simulink model "URController"  (R2023a)
settings: Solver=ode4  StartTime=0.0  StopTime=3  FixedStep=0.001  RelTol=1e-3  EnableMultiTasking=on
values from neighbouring files (symbols this model uses):
  CYCLE_FREQ = 0.001    [init.m]
  MAX_ACC = 100    [init.m]
  MAX_VEL = 180    [init.m]
libraries: slpidlib x13, forwardkinematics x2, simulink x1
(part 2 of 3)

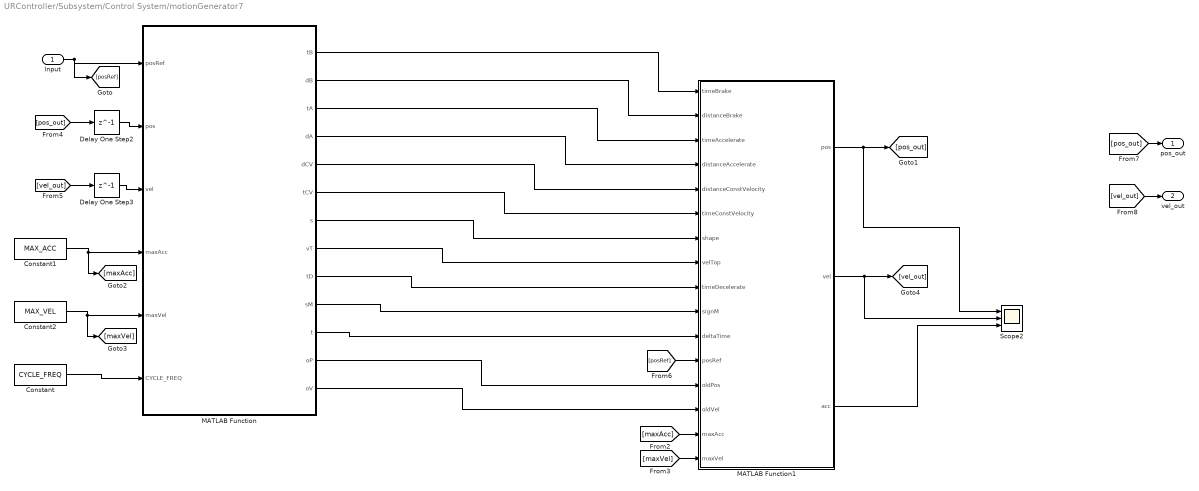
== system URController/Subsystem/Control System/motionGenerator7 ==
  Input : Inport
  Constant : Constant  Value=CYCLE_FREQ
  Constant1 : Constant  Value=MAX_ACC
  Constant2 : Constant  Value=MAX_VEL
  Delay One Step2 : Delay  DelayLength=1
  Delay One Step3 : Delay  DelayLength=1
  MATLAB Function : MATLAB Function  TreatAsAtomicUnit=on
  MATLAB Function1 : MATLAB Function  TreatAsAtomicUnit=on
  Scope2 : Scope  NumInputPorts=3
  pos_out : Outport
  vel_out : Outport  Port=2
  wires:
  [vel_out] -> Delay One Step3/1
  Delay One Step3/1 -> MATLAB Function/3(vel)
  MATLAB Function/9(tD) -> MATLAB Function1/9(timeDecelerate)
  Constant2/1 -> [maxVel], MATLAB Function/5(maxVel)
  MATLAB Function/5(dCV) -> MATLAB Function1/5(distanceConstVelocity)
  [pos_out] -> Delay One Step2/1
  MATLAB Function/8(vT) -> MATLAB Function1/8(velTop)
  MATLAB Function/2(dB) -> MATLAB Function1/2(distanceBrake)
  MATLAB Function1/2(vel) -> Scope2/2, [vel_out]
  Constant1/1 -> [maxAcc], MATLAB Function/4(maxAcc)
  [maxAcc] -> MATLAB Function1/15(maxAcc)
  MATLAB Function/1(tB) -> MATLAB Function1/1(timeBrake)
  MATLAB Function1/1(pos) -> Scope2/1, [pos_out]
  MATLAB Function/11(t) -> MATLAB Function1/11(deltaTime)
  Delay One Step2/1 -> MATLAB Function/2(pos)
  MATLAB Function/7(s) -> MATLAB Function1/7(shape)
  MATLAB Function/10(sM) -> MATLAB Function1/10(signM)
  MATLAB Function/6(tCV) -> MATLAB Function1/6(timeConstVelocity)
  Input/1 -> [posRef], MATLAB Function/1(posRef)
  [maxVel] -> MATLAB Function1/16(maxVel)
  MATLAB Function/4(dA) -> MATLAB Function1/4(distanceAccelerate)
  MATLAB Function/3(tA) -> MATLAB Function1/3(timeAccelerate)
  [posRef] -> MATLAB Function1/12(posRef)
  MATLAB Function1/3(acc) -> Scope2/3
  [pos_out] -> pos_out/1
  [vel_out] -> vel_out/1
  Constant/1 -> MATLAB Function/6(CYCLE_FREQ)
  MATLAB Function/12(oP) -> MATLAB Function1/13(oldPos)
  MATLAB Function/13(oV) -> MATLAB Function1/14(oldVel)

== matlab function URController/Subsystem/Control System/motionGenerator2/MATLAB Function ==
  settings: updateMethod=DISCRETE
  data: posRef input; pos input; vel input; tB output; maxAcc input; maxVel input; dB output; tA output; dA output; dCV output; tCV output; s output; vT output; tD output; sM output; t output; CYCLE_FREQ input; oP output; oV output
% oldPose: initial 0 and loop with output pos
% oldvel: initial 0 and loop with output vel

function [tB, dB, tA, dA, dCV, tCV, s, vT, tD, sM, t, oP, oV] = motionGenerator(posRef, pos, vel, maxAcc, maxVel, CYCLE_FREQ)
    persistent timeBrake distanceBrake;
    persistent timeAccelerate distanceAccelerate;
    persistent distanceConstVelocity timeConstVelocity;
    persistent timeDecelerate;
    persistent shape velTop signM;
    persistent oldPoseRef oldPos oldVel;
    persistent time;
    
    % Initialize the first time the function is called
    if (isempty(timeBrake) || isempty(distanceBrake) || isempty(timeAccelerate) || isempty(distanceAccelerate) ...
            || isempty(distanceConstVelocity) || isempty(timeConstVelocity) || isempty(timeDecelerate) ...
            || isempty(shape) || isempty(velTop) || isempty(signM) || isempty(oldPoseRef) || isempty(oldPos) ...
            || isempty(oldVel) || isempty(time))
        timeBrake = 0;
        distanceBrake = 0;
        timeAccelerate = 0;
        distanceAccelerate = 0;
        distanceConstVelocity = 0;
        timeConstVelocity = 0;
        timeDecelerate = 0;
        shape = 0;
        velTop = 0;
        signM = 0;
        oldPoseRef = 0;
        oldPos = 0;
        oldVel = 0;
        time = 0;

        tB = timeBrake;
        dB = distanceBrake;
        tA = timeAccelerate;
        dA = distanceAccelerate;
        dCV = distanceConstVelocity;
        tCV = timeConstVelocity;
        tD = timeDecelerate;
        s = shape;
        vT = velTop;
        sM = signM;
        t = time;
        oV = oldVel;
        oP = oldPos;
        return;
    end
    
    if (oldPoseRef ~= posRef)
        oldPos = pos;
        oldVel = vel;
        oldPoseRef = posRef;
        time = 0;

        tB = abs(oldVel) / maxAcc;
        dB = tB * abs(oldVel) / 2;
    
        sM = sign(posRef - (oldPos + sign(oldVel)*dB));
        
        if (sM ~= sign(oldVel))  % means brake is needed
            tA = (maxVel / maxAcc);
            dA = tA * (maxVel / 2);
        else
            tB = 0;
            dB = 0;
            tA = (maxVel - abs(oldVel)) / maxAcc;
            dA = tA * (maxVel + abs(oldVel)) / 2;
        end
    
        distanceTotal = abs(posRef - oldPos + sM*dB);
                    
        tD = maxVel / maxAcc;
        distanceDecelerate = tD * (maxVel) / 2;
        dCV = distanceTotal - (dA + distanceDecelerate);
        tCV = dCV / maxVel;
    
        if (tCV > 0)    % trapezoidal s
            s = 1;
            vT = 0;
        else                % triangular s
            s = 0;
            % Recalculate distances and periods
            if (sM ~= sign(oldVel))  % means brake is needed
                vT = sqrt(maxAcc*(distanceTotal));
                tA = (vT / maxAcc);
                dA = tA * (vT / 2);
            else
                tB = 0;
                dB = 0;
                distanceTotal = abs(posRef - oldPos);      % recalculate total distance
                vT = sqrt(0.5*oldVel^2 + maxAcc*distanceTotal);
                tA = (vT - abs(oldVel)) / maxAcc;
                dA = tA * (vT + abs(oldVel)) / 2;
            end
            tD = vT / maxAcc;
            distanceDecelerate = tD * (vT) / 2;
        end
        timeBrake = tB;
        distanceBrake = dB;
        timeAccelerate = tA;
        distanceAccelerate = dA;
        distanceConstVelocity = dCV;
        timeConstVelocity = tCV;
        timeDecelerate = tD;
        shape = s;
        velTop = vT;
        signM = sM;
        oV = oldVel;
        oP = oldPos;
    end
    
    tB = timeBrake;
    dB = distanceBrake;
    tA = timeAccelerate;
    dA = distanceAccelerate;
    dCV = distanceConstVelocity;
    tCV = timeConstVelocity;
    tD = timeDecelerate;
    s = shape;
    vT = velTop;
    sM = signM;
    time = time + CYCLE_FREQ;
    t = time;
    oV = oldVel;
    oP = oldPos;
end

== matlab function URController/Subsystem/Control System/motionGenerator2/MATLAB Function1 ==
  data: timeBrake input; distanceBrake input; timeAccelerate input; distanceAccelerate input; distanceConstVelocity input; timeConstVelocity input; shape input; velTop input; timeDecelerate input; signM input; deltaTime input; posRef input; pos output; vel output; oldPos input; oldVel input; maxAcc input; maxVel input; acc output
function [pos, vel, acc]   = calculateTrapezoidalProfile(timeBrake, distanceBrake, timeAccelerate, ...
    distanceAccelerate, distanceConstVelocity, timeConstVelocity, shape,  velTop, timeDecelerate, ...
    signM, deltaTime, posRef, oldPos, oldVel, maxAcc, maxVel)
    
    t = deltaTime;
    acc = 0;
    
    if (shape)   % trapezoidal shape
        if (t <= (timeBrake+timeAccelerate))
            pos = oldPos + oldVel*t + signM * 0.5*maxAcc*t^2;
            vel = oldVel + signM * maxAcc*t;
            acc = signM * maxAcc;
        elseif (t > (timeBrake+timeAccelerate) && t < (timeBrake+timeAccelerate+timeConstVelocity))
            pos = oldPos + signM * (-distanceBrake + distanceAccelerate + maxVel*(t-timeBrake-timeAccelerate));
            vel = signM * maxVel;
            % MG.acc = 0;
        elseif (t >= (timeBrake+timeAccelerate+timeConstVelocity) && t < (timeBrake+timeAccelerate+timeConstVelocity+timeDecelerate))
            pos = oldPos + signM * (-distanceBrake + distanceAccelerate + distanceConstVelocity + maxVel*(t-timeBrake-timeAccelerate-timeConstVelocity) - 0.5*maxAcc*(t-timeBrake-timeAccelerate-timeConstVelocity)^2);
            vel = signM * (maxVel - maxAcc*(t-timeBrake-timeAccelerate-timeConstVelocity));
            acc = - signM * maxAcc;
        else
            pos = posRef;
            vel = 0;
            % MG.acc = 0;
        end
    else            % triangular shape
        if (t <= (timeBrake+timeAccelerate))
            pos = oldPos + oldVel*t + signM * 0.5*maxAcc*t^2;
            vel = oldVel + signM * maxAcc*t;
            acc = signM * maxAcc;
        elseif (t > (timeBrake+timeAccelerate) && t < (timeBrake+timeAccelerate+timeDecelerate))
            pos = oldPos + signM * (-distanceBrake + distanceAccelerate + velTop*(t-timeBrake-timeAccelerate) - 0.5*maxAcc*(t-timeBrake-timeAccelerate)^2);
            vel = signM * (velTop - maxAcc*(t-timeBrake-timeAccelerate));
            acc = - signM * maxAcc;
        else
            pos = posRef;
            vel = 0;
            acc = 0;
        end
        
    end

end

== matlab function URController/Subsystem/Control System/motionGenerator3/MATLAB Function ==
  settings: updateMethod=DISCRETE
  data: posRef input; pos input; vel input; tB output; maxAcc input; maxVel input; dB output; tA output; dA output; dCV output; tCV output; s output; vT output; tD output; sM output; t output; CYCLE_FREQ input; oP output; oV output
% oldPose: initial 0 and loop with output pos
% oldvel: initial 0 and loop with output vel

function [tB, dB, tA, dA, dCV, tCV, s, vT, tD, sM, t, oP, oV] = motionGenerator(posRef, pos, vel, maxAcc, maxVel, CYCLE_FREQ)
    persistent timeBrake distanceBrake;
    persistent timeAccelerate distanceAccelerate;
    persistent distanceConstVelocity timeConstVelocity;
    persistent timeDecelerate;
    persistent shape velTop signM;
    persistent oldPoseRef oldPos oldVel;
    persistent time;
    
    % Initialize the first time the function is called
    if (isempty(timeBrake) || isempty(distanceBrake) || isempty(timeAccelerate) || isempty(distanceAccelerate) ...
            || isempty(distanceConstVelocity) || isempty(timeConstVelocity) || isempty(timeDecelerate) ...
            || isempty(shape) || isempty(velTop) || isempty(signM) || isempty(oldPoseRef) || isempty(oldPos) ...
            || isempty(oldVel) || isempty(time))
        timeBrake = 0;
        distanceBrake = 0;
        timeAccelerate = 0;
        distanceAccelerate = 0;
        distanceConstVelocity = 0;
        timeConstVelocity = 0;
        timeDecelerate = 0;
        shape = 0;
        velTop = 0;
        signM = 0;
        oldPoseRef = 0;
        oldPos = 0;
        oldVel = 0;
        time = 0;

        tB = timeBrake;
        dB = distanceBrake;
        tA = timeAccelerate;
        dA = distanceAccelerate;
        dCV = distanceConstVelocity;
        tCV = timeConstVelocity;
        tD = timeDecelerate;
        s = shape;
        vT = velTop;
        sM = signM;
        t = time;
        oV = oldVel;
        oP = oldPos;
        return;
    end
    
    if (oldPoseRef ~= posRef)
        oldPos = pos;
        oldVel = vel;
        oldPoseRef = posRef;
        time = 0;

        tB = abs(oldVel) / maxAcc;
        dB = tB * abs(oldVel) / 2;
    
        sM = sign(posRef - (oldPos + sign(oldVel)*dB));
        
        if (sM ~= sign(oldVel))  % means brake is needed
            tA = (maxVel / maxAcc);
            dA = tA * (maxVel / 2);
        else
            tB = 0;
            dB = 0;
            tA = (maxVel - abs(oldVel)) / maxAcc;
            dA = tA * (maxVel + abs(oldVel)) / 2;
        end
    
        distanceTotal = abs(posRef - oldPos + sM*dB);
                    
        tD = maxVel / maxAcc;
        distanceDecelerate = tD * (maxVel) / 2;
        dCV = distanceTotal - (dA + distanceDecelerate);
        tCV = dCV / maxVel;
    
        if (tCV > 0)    % trapezoidal s
            s = 1;
            vT = 0;
        else                % triangular s
            s = 0;
            % Recalculate distances and periods
            if (sM ~= sign(oldVel))  % means brake is needed
                vT = sqrt(maxAcc*(distanceTotal));
                tA = (vT / maxAcc);
                dA = tA * (vT / 2);
            else
                tB = 0;
                dB = 0;
                distanceTotal = abs(posRef - oldPos);      % recalculate total distance
                vT = sqrt(0.5*oldVel^2 + maxAcc*distanceTotal);
                tA = (vT - abs(oldVel)) / maxAcc;
                dA = tA * (vT + abs(oldVel)) / 2;
            end
            tD = vT / maxAcc;
            distanceDecelerate = tD * (vT) / 2;
        end
        timeBrake = tB;
        distanceBrake = dB;
        timeAccelerate = tA;
        distanceAccelerate = dA;
        distanceConstVelocity = dCV;
        timeConstVelocity = tCV;
        timeDecelerate = tD;
        shape = s;
        velTop = vT;
        signM = sM;
        oV = oldVel;
        oP = oldPos;
    end
    
    tB = timeBrake;
    dB = distanceBrake;
    tA = timeAccelerate;
    dA = distanceAccelerate;
    dCV = distanceConstVelocity;
    tCV = timeConstVelocity;
    tD = timeDecelerate;
    s = shape;
    vT = velTop;
    sM = signM;
    time = time + CYCLE_FREQ;
    t = time;
    oV = oldVel;
    oP = oldPos;
end

== matlab function URController/Subsystem/Control System/motionGenerator3/MATLAB Function1 ==
  data: timeBrake input; distanceBrake input; timeAccelerate input; distanceAccelerate input; distanceConstVelocity input; timeConstVelocity input; shape input; velTop input; timeDecelerate input; signM input; deltaTime input; posRef input; pos output; vel output; oldPos input; oldVel input; maxAcc input; maxVel input; acc output
function [pos, vel, acc]   = calculateTrapezoidalProfile(timeBrake, distanceBrake, timeAccelerate, ...
    distanceAccelerate, distanceConstVelocity, timeConstVelocity, shape,  velTop, timeDecelerate, ...
    signM, deltaTime, posRef, oldPos, oldVel, maxAcc, maxVel)
    
    t = deltaTime;
    acc = 0;
    
    if (shape)   % trapezoidal shape
        if (t <= (timeBrake+timeAccelerate))
            pos = oldPos + oldVel*t + signM * 0.5*maxAcc*t^2;
            vel = oldVel + signM * maxAcc*t;
            acc = signM * maxAcc;
        elseif (t > (timeBrake+timeAccelerate) && t < (timeBrake+timeAccelerate+timeConstVelocity))
            pos = oldPos + signM * (-distanceBrake + distanceAccelerate + maxVel*(t-timeBrake-timeAccelerate));
            vel = signM * maxVel;
            % MG.acc = 0;
        elseif (t >= (timeBrake+timeAccelerate+timeConstVelocity) && t < (timeBrake+timeAccelerate+timeConstVelocity+timeDecelerate))
            pos = oldPos + signM * (-distanceBrake + distanceAccelerate + distanceConstVelocity + maxVel*(t-timeBrake-timeAccelerate-timeConstVelocity) - 0.5*maxAcc*(t-timeBrake-timeAccelerate-timeConstVelocity)^2);
            vel = signM * (maxVel - maxAcc*(t-timeBrake-timeAccelerate-timeConstVelocity));
            acc = - signM * maxAcc;
        else
            pos = posRef;
            vel = 0;
            % MG.acc = 0;
        end
    else            % triangular shape
        if (t <= (timeBrake+timeAccelerate))
            pos = oldPos + oldVel*t + signM * 0.5*maxAcc*t^2;
            vel = oldVel + signM * maxAcc*t;
            acc = signM * maxAcc;
        elseif (t > (timeBrake+timeAccelerate) && t < (timeBrake+timeAccelerate+timeDecelerate))
            pos = oldPos + signM * (-distanceBrake + distanceAccelerate + velTop*(t-timeBrake-timeAccelerate) - 0.5*maxAcc*(t-timeBrake-timeAccelerate)^2);
            vel = signM * (velTop - maxAcc*(t-timeBrake-timeAccelerate));
            acc = - signM * maxAcc;
        else
            pos = posRef;
            vel = 0;
            acc = 0;
        end
        
    end

end

== matlab function URController/Subsystem/Control System/motionGenerator4/MATLAB Function ==
  settings: updateMethod=DISCRETE
  data: posRef input; pos input; vel input; tB output; maxAcc input; maxVel input; dB output; tA output; dA output; dCV output; tCV output; s output; vT output; tD output; sM output; t output; CYCLE_FREQ input; oP output; oV output
% oldPose: initial 0 and loop with output pos
% oldvel: initial 0 and loop with output vel

function [tB, dB, tA, dA, dCV, tCV, s, vT, tD, sM, t, oP, oV] = motionGenerator(posRef, pos, vel, maxAcc, maxVel, CYCLE_FREQ)
    persistent timeBrake distanceBrake;
    persistent timeAccelerate distanceAccelerate;
    persistent distanceConstVelocity timeConstVelocity;
    persistent timeDecelerate;
    persistent shape velTop signM;
    persistent oldPoseRef oldPos oldVel;
    persistent time;
    
    % Initialize the first time the function is called
    if (isempty(timeBrake) || isempty(distanceBrake) || isempty(timeAccelerate) || isempty(distanceAccelerate) ...
            || isempty(distanceConstVelocity) || isempty(timeConstVelocity) || isempty(timeDecelerate) ...
            || isempty(shape) || isempty(velTop) || isempty(signM) || isempty(oldPoseRef) || isempty(oldPos) ...
            || isempty(oldVel) || isempty(time))
        timeBrake = 0;
        distanceBrake = 0;
        timeAccelerate = 0;
        distanceAccelerate = 0;
        distanceConstVelocity = 0;
        timeConstVelocity = 0;
        timeDecelerate = 0;
        shape = 0;
        velTop = 0;
        signM = 0;
        oldPoseRef = 0;
        oldPos = 0;
        oldVel = 0;
        time = 0;

        tB = timeBrake;
        dB = distanceBrake;
        tA = timeAccelerate;
        dA = distanceAccelerate;
        dCV = distanceConstVelocity;
        tCV = timeConstVelocity;
        tD = timeDecelerate;
        s = shape;
        vT = velTop;
        sM = signM;
        t = time;
        oV = oldVel;
        oP = oldPos;
        return;
    end
    
    if (oldPoseRef ~= posRef)
        oldPos = pos;
        oldVel = vel;
        oldPoseRef = posRef;
        time = 0;

        tB = abs(oldVel) / maxAcc;
        dB = tB * abs(oldVel) / 2;
    
        sM = sign(posRef - (oldPos + sign(oldVel)*dB));
        
        if (sM ~= sign(oldVel))  % means brake is needed
            tA = (maxVel / maxAcc);
            dA = tA * (maxVel / 2);
        else
            tB = 0;
            dB = 0;
            tA = (maxVel - abs(oldVel)) / maxAcc;
            dA = tA * (maxVel + abs(oldVel)) / 2;
        end
    
        distanceTotal = abs(posRef - oldPos + sM*dB);
                    
        tD = maxVel / maxAcc;
        distanceDecelerate = tD * (maxVel) / 2;
        dCV = distanceTotal - (dA + distanceDecelerate);
        tCV = dCV / maxVel;
    
        if (tCV > 0)    % trapezoidal s
            s = 1;
            vT = 0;
        else                % triangular s
            s = 0;
            % Recalculate distances and periods
            if (sM ~= sign(oldVel))  % means brake is needed
                vT = sqrt(maxAcc*(distanceTotal));
                tA = (vT / maxAcc);
                dA = tA * (vT / 2);
            else
                tB = 0;
                dB = 0;
                distanceTotal = abs(posRef - oldPos);      % recalculate total distance
                vT = sqrt(0.5*oldVel^2 + maxAcc*distanceTotal);
                tA = (vT - abs(oldVel)) / maxAcc;
                dA = tA * (vT + abs(oldVel)) / 2;
            end
            tD = vT / maxAcc;
            distanceDecelerate = tD * (vT) / 2;
        end
        timeBrake = tB;
        distanceBrake = dB;
        timeAccelerate = tA;
        distanceAccelerate = dA;
        distanceConstVelocity = dCV;
        timeConstVelocity = tCV;
        timeDecelerate = tD;
        shape = s;
        velTop = vT;
        signM = sM;
        oV = oldVel;
        oP = oldPos;
    end
    
    tB = timeBrake;
    dB = distanceBrake;
    tA = timeAccelerate;
    dA = distanceAccelerate;
    dCV = distanceConstVelocity;
    tCV = timeConstVelocity;
    tD = timeDecelerate;
    s = shape;
    vT = velTop;
    sM = signM;
    time = time + CYCLE_FREQ;
    t = time;
    oV = oldVel;
    oP = oldPos;
end

== matlab function URController/Subsystem/Control System/motionGenerator4/MATLAB Function1 ==
  data: timeBrake input; distanceBrake input; timeAccelerate input; distanceAccelerate input; distanceConstVelocity input; timeConstVelocity input; shape input; velTop input; timeDecelerate input; signM input; deltaTime input; posRef input; pos output; vel output; oldPos input; oldVel input; maxAcc input; maxVel input; acc output
function [pos, vel, acc]   = calculateTrapezoidalProfile(timeBrake, distanceBrake, timeAccelerate, ...
    distanceAccelerate, distanceConstVelocity, timeConstVelocity, shape,  velTop, timeDecelerate, ...
    signM, deltaTime, posRef, oldPos, oldVel, maxAcc, maxVel)
    
    t = deltaTime;
    acc = 0;
    
    if (shape)   % trapezoidal shape
        if (t <= (timeBrake+timeAccelerate))
            pos = oldPos + oldVel*t + signM * 0.5*maxAcc*t^2;
            vel = oldVel + signM * maxAcc*t;
            acc = signM * maxAcc;
        elseif (t > (timeBrake+timeAccelerate) && t < (timeBrake+timeAccelerate+timeConstVelocity))
            pos = oldPos + signM * (-distanceBrake + distanceAccelerate + maxVel*(t-timeBrake-timeAccelerate));
            vel = signM * maxVel;
            % MG.acc = 0;
        elseif (t >= (timeBrake+timeAccelerate+timeConstVelocity) && t < (timeBrake+timeAccelerate+timeConstVelocity+timeDecelerate))
            pos = oldPos + signM * (-distanceBrake + distanceAccelerate + distanceConstVelocity + maxVel*(t-timeBrake-timeAccelerate-timeConstVelocity) - 0.5*maxAcc*(t-timeBrake-timeAccelerate-timeConstVelocity)^2);
            vel = signM * (maxVel - maxAcc*(t-timeBrake-timeAccelerate-timeConstVelocity));
            acc = - signM * maxAcc;
        else
            pos = posRef;
            vel = 0;
            % MG.acc = 0;
        end
    else            % triangular shape
        if (t <= (timeBrake+timeAccelerate))
            pos = oldPos + oldVel*t + signM * 0.5*maxAcc*t^2;
            vel = oldVel + signM * maxAcc*t;
            acc = signM * maxAcc;
        elseif (t > (timeBrake+timeAccelerate) && t < (timeBrake+timeAccelerate+timeDecelerate))
            pos = oldPos + signM * (-distanceBrake + distanceAccelerate + velTop*(t-timeBrake-timeAccelerate) - 0.5*maxAcc*(t-timeBrake-timeAccelerate)^2);
            vel = signM * (velTop - maxAcc*(t-timeBrake-timeAccelerate));
            acc = - signM * maxAcc;
        else
            pos = posRef;
            vel = 0;
            acc = 0;
        end
        
    end

end

== matlab function URController/Subsystem/Control System/motionGenerator5/MATLAB Function ==
  settings: updateMethod=DISCRETE
  data: posRef input; pos input; vel input; tB output; maxAcc input; maxVel input; dB output; tA output; dA output; dCV output; tCV output; s output; vT output; tD output; sM output; t output; CYCLE_FREQ input; oP output; oV output
% oldPose: initial 0 and loop with output pos
% oldvel: initial 0 and loop with output vel

function [tB, dB, tA, dA, dCV, tCV, s, vT, tD, sM, t, oP, oV] = motionGenerator(posRef, pos, vel, maxAcc, maxVel, CYCLE_FREQ)
    persistent timeBrake distanceBrake;
    persistent timeAccelerate distanceAccelerate;
    persistent distanceConstVelocity timeConstVelocity;
    persistent timeDecelerate;
    persistent shape velTop signM;
    persistent oldPoseRef oldPos oldVel;
    persistent time;
    
    % Initialize the first time the function is called
    if (isempty(timeBrake) || isempty(distanceBrake) || isempty(timeAccelerate) || isempty(distanceAccelerate) ...
            || isempty(distanceConstVelocity) || isempty(timeConstVelocity) || isempty(timeDecelerate) ...
            || isempty(shape) || isempty(velTop) || isempty(signM) || isempty(oldPoseRef) || isempty(oldPos) ...
            || isempty(oldVel) || isempty(time))
        timeBrake = 0;
        distanceBrake = 0;
        timeAccelerate = 0;
        distanceAccelerate = 0;
        distanceConstVelocity = 0;
        timeConstVelocity = 0;
        timeDecelerate = 0;
        shape = 0;
        velTop = 0;
        signM = 0;
        oldPoseRef = 0;
        oldPos = 0;
        oldVel = 0;
        time = 0;

        tB = timeBrake;
        dB = distanceBrake;
        tA = timeAccelerate;
        dA = distanceAccelerate;
        dCV = distanceConstVelocity;
        tCV = timeConstVelocity;
        tD = timeDecelerate;
        s = shape;
        vT = velTop;
        sM = signM;
        t = time;
        oV = oldVel;
        oP = oldPos;
        return;
    end
    
    if (oldPoseRef ~= posRef)
        oldPos = pos;
        oldVel = vel;
        oldPoseRef = posRef;
        time = 0;

        tB = abs(oldVel) / maxAcc;
        dB = tB * abs(oldVel) / 2;
    
        sM = sign(posRef - (oldPos + sign(oldVel)*dB));
        
        if (sM ~= sign(oldVel))  % means brake is needed
            tA = (maxVel / maxAcc);
            dA = tA * (maxVel / 2);
        else
            tB = 0;
            dB = 0;
            tA = (maxVel - abs(oldVel)) / maxAcc;
            dA = tA * (maxVel + abs(oldVel)) / 2;
        end
    
        distanceTotal = abs(posRef - oldPos + sM*dB);
                    
        tD = maxVel / maxAcc;
        distanceDecelerate = tD * (maxVel) / 2;
        dCV = distanceTotal - (dA + distanceDecelerate);
        tCV = dCV / maxVel;
    
        if (tCV > 0)    % trapezoidal s
            s = 1;
            vT = 0;
        else                % triangular s
            s = 0;
            % Recalculate distances and periods
            if (sM ~= sign(oldVel))  % means brake is needed
                vT = sqrt(maxAcc*(distanceTotal));
                tA = (vT / maxAcc);
                dA = tA * (vT / 2);
            else
                tB = 0;
                dB = 0;
                distanceTotal = abs(posRef - oldPos);      % recalculate total distance
                vT = sqrt(0.5*oldVel^2 + maxAcc*distanceTotal);
                tA = (vT - abs(oldVel)) / maxAcc;
                dA = tA * (vT + abs(oldVel)) / 2;
            end
            tD = vT / maxAcc;
            distanceDecelerate = tD * (vT) / 2;
        end
        timeBrake = tB;
        distanceBrake = dB;
        timeAccelerate = tA;
        distanceAccelerate = dA;
        distanceConstVelocity = dCV;
        timeConstVelocity = tCV;
        timeDecelerate = tD;
        shape = s;
        velTop = vT;
        signM = sM;
        oV = oldVel;
        oP = oldPos;
    end
    
    tB = timeBrake;
    dB = distanceBrake;
    tA = timeAccelerate;
    dA = distanceAccelerate;
    dCV = distanceConstVelocity;
    tCV = timeConstVelocity;
    tD = timeDecelerate;
    s = shape;
    vT = velTop;
    sM = signM;
    time = time + CYCLE_FREQ;
    t = time;
    oV = oldVel;
    oP = oldPos;
end

== matlab function URController/Subsystem/Kinematic calculator/MATLAB Function ==
  data: gd input; theta output
function theta   = ur5InvKin( gd )
%%%%%%%%%%%%%%%%%%%%%%%%%%%%%%%%%%%%%%%%%%%%%%%
%%%%%%%%%%%%%%%%%%%% UR5INV %%%%%%%%%%%%%%%%%%%
%%%%%%%%%%%%%%%%%%%%%%%%%%%%%%%%%%%%%%%%%%%%%%%
%   Inverse kinematics of UR5
%   Formulas adapted from Ryan Keating's "UR5 Inverse Kinematics" paper
%   Input args:
%           gd - the 4x4 matrix - desired transformation from base to end
%   Output args:
%           theta - 6x8 matrix, each colum represents one possible solution 
%           of joint angles
    
    % Check input size
    if ~isequal(size(gd), [4,4])
        msg ='ur5invKin function: Wrong input format, must be a 4x4 matrix';
        error(msg);
    end

    theta = zeros(6, 8);
    % DH parameters
    d1 = 0.0892;
    d2 = 0;
    d3 = 0;
    d4 = 0.1093;
    d5 = 0.09475;
    d6 = 0.0825;
    a1 = 0;
    a2 = -0.425;
    a3 = -0.392;
    a4 = 0;
    a5 = 0;
    a6 = 0;
    alpha1 = pi/2;
    alpha2 = 0;
    alpha3 = 0;
    alpha4 = pi/2;
    alpha5 = -pi/2;
    alpha6 = 0;

    % Calculating theta1
    p05 = gd * [0, 0, -d6, 1]'  - [0, 0, 0, 1]';
    psi = atan2(p05(2), p05(1));
    phi = acos(d4 / sqrt(p05(2)*p05(2) + p05(1)*p05(1)));
    theta(1, 1:4) = pi/2 + psi + phi;
    theta(1, 5:8) = pi/2 + psi - phi;
    theta = real(theta);


    % Calculating theta5
    cols = [1, 5];
    for i=1:length(cols)
        c = cols(i);
        T10 = inv(DH(a1, alpha1, d1, theta(1,c)));
        T16 = T10 * gd;
        p16z = T16(3,4);
        t5 = acos((p16z-d4)/d6);
        theta(5, c:c+1) = t5;
        theta(5, c+2:c+3) = -t5;
    end
    theta = real(theta);

    % Calculating theta6
    cols = [1, 3, 5, 7];
    for i=1:length(cols)
        c = cols(i);
        T01 = DH(a1, alpha1, d1, theta(1,c));
        T61 = inv(gd) * T01;
        T61zy = T61(2, 3);
        T61zx = T61(1, 3);
        t5 = theta(5, c);
        theta(6, c:c+1) = atan2(-T61zy/sin(t5), T61zx/sin(t5));
    end
    theta = real(theta);

    % Calculating theta3
    cols = [1, 3, 5, 7];
    for i=1:length(cols)
        c = cols(i);
        T10 = inv(DH(a1, alpha1, d1, theta(1,c)));
        T65 = inv(DH(a6, alpha6, d6, theta(6,c)));
        T54 = inv(DH(a5, alpha5, d5, theta(5,c)));
        T14 = T10 * gd * T65 * T54;
        p13 = T14 * [0, -d4, 0, 1]' - [0,0,0,1]';
        p13norm2 = norm(p13) ^ 2;
        % disp((p13norm2-a2*a2-a3*a3)/(2*a2*a3));
        t3p = acos((p13norm2-a2*a2-a3*a3)/(2*a2*a3));
        theta(3, c) = t3p;
        theta(3, c+1) = -t3p;
    end
    theta = real(theta);

    % Calculating theta2 and theta4
    cols = [1, 2, 3, 4, 5, 6, 7, 8];
    for i=1:length(cols)
        c = cols(i);
        T10 = inv(DH(a1, alpha1, d1, theta(1,c)));
        T65 = inv(DH(a6, alpha6, d6, theta(6,c)));
        T54 = inv(DH(a5, alpha5, d5, theta(5,c)));
        T14 = T10 * gd * T65 * T54;
        p13 = T14 * [0, -d4, 0, 1]' - [0,0,0,1]';
        p13norm = norm(p13);
        theta(2, c) = -atan2(p13(2), -p13(1))+asin(a3*sin(theta(3,c))/p13norm);
        T32 = inv(DH(a3, alpha3, d3, theta(3,c)));
        T21 = inv(DH(a2, alpha2, d2, theta(2,c)));
        T34 = T32 * T21 * T14;
        theta(4, c) = atan2(T34(2,1), T34(1,1));
    end
    theta = real(theta);

    for j=1:8
        theta(1,j) = theta(1,j)-pi;
    end

    % Bound the joint angles from -pi to pi
    for i=1:6
        for j=1:8
            if theta(i,j) <= -pi
                theta(i,j) = theta(i,j) + 2*pi;
            elseif theta(i,j) > pi
                theta(i,j) = theta(i,j) - 2*pi;
            end
        end
    end
                
                    
end


% Function
% Params: roll value (radians) 
% Return: 3x3 rotation matrix

function rot_m33 = ROTX(roll)
    rot_m33 = [1 0 0 ; 0 cos(roll) -sin(roll); 0 sin(roll) cos(roll)];
end


% Function
% Params: yaw value (radians) 
% Return: 3x3 rotation matrix

function rot_m33 = ROTZ(yaw)
    rot_m33 = [cos(yaw) -sin(yaw) 0; sin(yaw) cos(yaw) 0; 0 0 1];
end

% Function
% Params: pitch value (radians) 
% Return: 3x3 rotation matrix

function rot_m33 = ROTY(pitch)
    rot_m33 = [cos(pitch) 0 sin(pitch) ; 0 1 0;-sin(pitch) 0 cos(pitch)];
end


function [ G ] = DH( a, alpha, d, theta )
%   Calculate transformation matrix from DH parameters
%   DH parameters follow the tranditional definition
    Td = eye(4);
    Td(3,4) = d;
    Ta = eye(4);
    Ta(1,4) = a;
    Rtheta = eye(4);
    Rtheta(1:3, 1:3) = ROTZ(theta);
    Ralpha = eye(4);
    Ralpha(1:3, 1:3) = ROTX(alpha);
    G = Td * Rtheta * Ta * Ralpha;
end

== matlab function URController/Subsystem/Control System/motionGenerator5/MATLAB Function1 ==
  data: timeBrake input; distanceBrake input; timeAccelerate input; distanceAccelerate input; distanceConstVelocity input; timeConstVelocity input; shape input; velTop input; timeDecelerate input; signM input; deltaTime input; posRef input; pos output; vel output; oldPos input; oldVel input; maxAcc input; maxVel input; acc output
function [pos, vel, acc]   = calculateTrapezoidalProfile(timeBrake, distanceBrake, timeAccelerate, ...
    distanceAccelerate, distanceConstVelocity, timeConstVelocity, shape,  velTop, timeDecelerate, ...
    signM, deltaTime, posRef, oldPos, oldVel, maxAcc, maxVel)
    
    t = deltaTime;
    acc = 0;
    
    if (shape)   % trapezoidal shape
        if (t <= (timeBrake+timeAccelerate))
            pos = oldPos + oldVel*t + signM * 0.5*maxAcc*t^2;
            vel = oldVel + signM * maxAcc*t;
            acc = signM * maxAcc;
        elseif (t > (timeBrake+timeAccelerate) && t < (timeBrake+timeAccelerate+timeConstVelocity))
            pos = oldPos + signM * (-distanceBrake + distanceAccelerate + maxVel*(t-timeBrake-timeAccelerate));
            vel = signM * maxVel;
            % MG.acc = 0;
        elseif (t >= (timeBrake+timeAccelerate+timeConstVelocity) && t < (timeBrake+timeAccelerate+timeConstVelocity+timeDecelerate))
            pos = oldPos + signM * (-distanceBrake + distanceAccelerate + distanceConstVelocity + maxVel*(t-timeBrake-timeAccelerate-timeConstVelocity) - 0.5*maxAcc*(t-timeBrake-timeAccelerate-timeConstVelocity)^2);
            vel = signM * (maxVel - maxAcc*(t-timeBrake-timeAccelerate-timeConstVelocity));
            acc = - signM * maxAcc;
        else
            pos = posRef;
            vel = 0;
            % MG.acc = 0;
        end
    else            % triangular shape
        if (t <= (timeBrake+timeAccelerate))
            pos = oldPos + oldVel*t + signM * 0.5*maxAcc*t^2;
            vel = oldVel + signM * maxAcc*t;
            acc = signM * maxAcc;
        elseif (t > (timeBrake+timeAccelerate) && t < (timeBrake+timeAccelerate+timeDecelerate))
            pos = oldPos + signM * (-distanceBrake + distanceAccelerate + velTop*(t-timeBrake-timeAccelerate) - 0.5*maxAcc*(t-timeBrake-timeAccelerate)^2);
            vel = signM * (velTop - maxAcc*(t-timeBrake-timeAccelerate));
            acc = - signM * maxAcc;
        else
            pos = posRef;
            vel = 0;
            acc = 0;
        end
        
    end

end

== matlab function URController/Subsystem/Control System/motionGenerator7/MATLAB Function ==
  settings: updateMethod=DISCRETE
  data: posRef input; pos input; vel input; tB output; maxAcc input; maxVel input; dB output; tA output; dA output; dCV output; tCV output; s output; vT output; tD output; sM output; t output; CYCLE_FREQ input; oP output; oV output
% oldPose: initial 0 and loop with output pos
% oldvel: initial 0 and loop with output vel

function [tB, dB, tA, dA, dCV, tCV, s, vT, tD, sM, t, oP, oV] = motionGenerator(posRef, pos, vel, maxAcc, maxVel, CYCLE_FREQ)
    persistent timeBrake distanceBrake;
    persistent timeAccelerate distanceAccelerate;
    persistent distanceConstVelocity timeConstVelocity;
    persistent timeDecelerate;
    persistent shape velTop signM;
    persistent oldPoseRef oldPos oldVel;
    persistent time;
    
    % Initialize the first time the function is called
    if (isempty(timeBrake) || isempty(distanceBrake) || isempty(timeAccelerate) || isempty(distanceAccelerate) ...
            || isempty(distanceConstVelocity) || isempty(timeConstVelocity) || isempty(timeDecelerate) ...
            || isempty(shape) || isempty(velTop) || isempty(signM) || isempty(oldPoseRef) || isempty(oldPos) ...
            || isempty(oldVel) || isempty(time))
        timeBrake = 0;
        distanceBrake = 0;
        timeAccelerate = 0;
        distanceAccelerate = 0;
        distanceConstVelocity = 0;
        timeConstVelocity = 0;
        timeDecelerate = 0;
        shape = 0;
        velTop = 0;
        signM = 0;
        oldPoseRef = 0;
        oldPos = 0;
        oldVel = 0;
        time = 0;

        tB = timeBrake;
        dB = distanceBrake;
        tA = timeAccelerate;
        dA = distanceAccelerate;
        dCV = distanceConstVelocity;
        tCV = timeConstVelocity;
        tD = timeDecelerate;
        s = shape;
        vT = velTop;
        sM = signM;
        t = time;
        oV = oldVel;
        oP = oldPos;
        return;
    end
    
    if (oldPoseRef ~= posRef)
        oldPos = pos;
        oldVel = vel;
        oldPoseRef = posRef;
        time = 0;

        tB = abs(oldVel) / maxAcc;
        dB = tB * abs(oldVel) / 2;
    
        sM = sign(posRef - (oldPos + sign(oldVel)*dB));
        
        if (sM ~= sign(oldVel))  % means brake is needed
            tA = (maxVel / maxAcc);
            dA = tA * (maxVel / 2);
        else
            tB = 0;
            dB = 0;
            tA = (maxVel - abs(oldVel)) / maxAcc;
            dA = tA * (maxVel + abs(oldVel)) / 2;
        end
    
        distanceTotal = abs(posRef - oldPos + sM*dB);
                    
        tD = maxVel / maxAcc;
        distanceDecelerate = tD * (maxVel) / 2;
        dCV = distanceTotal - (dA + distanceDecelerate);
        tCV = dCV / maxVel;
    
        if (tCV > 0)    % trapezoidal s
            s = 1;
            vT = 0;
        else                % triangular s
            s = 0;
            % Recalculate distances and periods
            if (sM ~= sign(oldVel))  % means brake is needed
                vT = sqrt(maxAcc*(distanceTotal));
                tA = (vT / maxAcc);
                dA = tA * (vT / 2);
            else
                tB = 0;
                dB = 0;
                distanceTotal = abs(posRef - oldPos);      % recalculate total distance
                vT = sqrt(0.5*oldVel^2 + maxAcc*distanceTotal);
                tA = (vT - abs(oldVel)) / maxAcc;
                dA = tA * (vT + abs(oldVel)) / 2;
            end
            tD = vT / maxAcc;
            distanceDecelerate = tD * (vT) / 2;
        end
        timeBrake = tB;
        distanceBrake = dB;
        timeAccelerate = tA;
        distanceAccelerate = dA;
        distanceConstVelocity = dCV;
        timeConstVelocity = tCV;
        timeDecelerate = tD;
        shape = s;
        velTop = vT;
        signM = sM;
        oV = oldVel;
        oP = oldPos;
    end
    
    tB = timeBrake;
    dB = distanceBrake;
    tA = timeAccelerate;
    dA = distanceAccelerate;
    dCV = distanceConstVelocity;
    tCV = timeConstVelocity;
    tD = timeDecelerate;
    s = shape;
    vT = velTop;
    sM = signM;
    time = time + CYCLE_FREQ;
    t = time;
    oV = oldVel;
    oP = oldPos;
end

== matlab function URController/Subsystem/Control System/motionGenerator7/MATLAB Function1 ==
  data: timeBrake input; distanceBrake input; timeAccelerate input; distanceAccelerate input; distanceConstVelocity input; timeConstVelocity input; shape input; velTop input; timeDecelerate input; signM input; deltaTime input; posRef input; pos output; vel output; oldPos input; oldVel input; maxAcc input; maxVel input; acc output
function [pos, vel, acc]   = calculateTrapezoidalProfile(timeBrake, distanceBrake, timeAccelerate, ...
    distanceAccelerate, distanceConstVelocity, timeConstVelocity, shape,  velTop, timeDecelerate, ...
    signM, deltaTime, posRef, oldPos, oldVel, maxAcc, maxVel)
    
    t = deltaTime;
    acc = 0;
    
    if (shape)   % trapezoidal shape
        if (t <= (timeBrake+timeAccelerate))
            pos = oldPos + oldVel*t + signM * 0.5*maxAcc*t^2;
            vel = oldVel + signM * maxAcc*t;
            acc = signM * maxAcc;
        elseif (t > (timeBrake+timeAccelerate) && t < (timeBrake+timeAccelerate+timeConstVelocity))
            pos = oldPos + signM * (-distanceBrake + distanceAccelerate + maxVel*(t-timeBrake-timeAccelerate));
            vel = signM * maxVel;
            % MG.acc = 0;
        elseif (t >= (timeBrake+timeAccelerate+timeConstVelocity) && t < (timeBrake+timeAccelerate+timeConstVelocity+timeDecelerate))
            pos = oldPos + signM * (-distanceBrake + distanceAccelerate + distanceConstVelocity + maxVel*(t-timeBrake-timeAccelerate-timeConstVelocity) - 0.5*maxAcc*(t-timeBrake-timeAccelerate-timeConstVelocity)^2);
            vel = signM * (maxVel - maxAcc*(t-timeBrake-timeAccelerate-timeConstVelocity));
            acc = - signM * maxAcc;
        else
            pos = posRef;
            vel = 0;
            % MG.acc = 0;
        end
    else            % triangular shape
        if (t <= (timeBrake+timeAccelerate))
            pos = oldPos + oldVel*t + signM * 0.5*maxAcc*t^2;
            vel = oldVel + signM * maxAcc*t;
            acc = signM * maxAcc;
        elseif (t > (timeBrake+timeAccelerate) && t < (timeBrake+timeAccelerate+timeDecelerate))
            pos = oldPos + signM * (-distanceBrake + distanceAccelerate + velTop*(t-timeBrake-timeAccelerate) - 0.5*maxAcc*(t-timeBrake-timeAccelerate)^2);
            vel = signM * (velTop - maxAcc*(t-timeBrake-timeAccelerate));
            acc = - signM * maxAcc;
        else
            pos = posRef;
            vel = 0;
            acc = 0;
        end
        
    end

end

== matlab function URController/Subsystem/Kinematic calculator/MATLAB Function1 ==
  data: pos_orient_arr input; gd output
function gd = gdConverter(pos_orient_arr)

gd = eye(4);

for i = 1:3
    gd(i, 4) = pos_orient_arr(i);
end

rot_m33 = EULERXYZ(pos_orient_arr(4:6));

gd(1:3, 1:3) = rot_m33;

end

% Function
% Params: roll value (radians) 
% Return: 3x3 rotation matrix

function rot_m33 = ROTX(roll)
    rot_m33 = [1 0 0 ; 0 cos(roll) -sin(roll); 0 sin(roll) cos(roll)];
end


% Function
% Params: yaw value (radians) 
% Return: 3x3 rotation matrix

function rot_m33 = ROTZ(yaw)
    rot_m33 = [cos(yaw) -sin(yaw) 0; sin(yaw) cos(yaw) 0; 0 0 1];
end

% Function
% Params: pitch value (radians) 
% Return: 3x3 rotation matrix

function rot_m33 = ROTY(pitch)
    rot_m33 = [cos(pitch) 0 sin(pitch) ; 0 1 0;-sin(pitch) 0 cos(pitch)];
end


function [totalRot] = EULERXYZ( angles )
% multiplies rotation matrices of X, Y, Z axis

totalRot = ROTX(angles(1)) * ROTY(angles(2)) * ROTZ(angles(3));

end

== matlab function URController/Subsystem/Control System/motionGenerator6/MATLAB Function ==
  settings: updateMethod=DISCRETE
  data: posRef input; pos input; vel input; tB output; maxAcc input; maxVel input; dB output; tA output; dA output; dCV output; tCV output; s output; vT output; tD output; sM output; t output; CYCLE_FREQ input; oP output; oV output
% oldPose: initial 0 and loop with output pos
% oldvel: initial 0 and loop with output vel

function [tB, dB, tA, dA, dCV, tCV, s, vT, tD, sM, t, oP, oV] = motionGenerator(posRef, pos, vel, maxAcc, maxVel, CYCLE_FREQ)
    persistent timeBrake distanceBrake;
    persistent timeAccelerate distanceAccelerate;
    persistent distanceConstVelocity timeConstVelocity;
    persistent timeDecelerate;
    persistent shape velTop signM;
    persistent oldPoseRef oldPos oldVel;
    persistent time;
    
    % Initialize the first time the function is called
    if (isempty(timeBrake) || isempty(distanceBrake) || isempty(timeAccelerate) || isempty(distanceAccelerate) ...
            || isempty(distanceConstVelocity) || isempty(timeConstVelocity) || isempty(timeDecelerate) ...
            || isempty(shape) || isempty(velTop) || isempty(signM) || isempty(oldPoseRef) || isempty(oldPos) ...
            || isempty(oldVel) || isempty(time))
        timeBrake = 0;
        distanceBrake = 0;
        timeAccelerate = 0;
        distanceAccelerate = 0;
        distanceConstVelocity = 0;
        timeConstVelocity = 0;
        timeDecelerate = 0;
        shape = 0;
        velTop = 0;
        signM = 0;
        oldPoseRef = 0;
        oldPos = 0;
        oldVel = 0;
        time = 0;

        tB = timeBrake;
        dB = distanceBrake;
        tA = timeAccelerate;
        dA = distanceAccelerate;
        dCV = distanceConstVelocity;
        tCV = timeConstVelocity;
        tD = timeDecelerate;
        s = shape;
        vT = velTop;
        sM = signM;
        t = time;
        oV = oldVel;
        oP = oldPos;
        return;
    end
    
    if (oldPoseRef ~= posRef)
        oldPos = pos;
        oldVel = vel;
        oldPoseRef = posRef;
        time = 0;

        tB = abs(oldVel) / maxAcc;
        dB = tB * abs(oldVel) / 2;
    
        sM = sign(posRef - (oldPos + sign(oldVel)*dB));
        
        if (sM ~= sign(oldVel))  % means brake is needed
            tA = (maxVel / maxAcc);
            dA = tA * (maxVel / 2);
        else
            tB = 0;
            dB = 0;
            tA = (maxVel - abs(oldVel)) / maxAcc;
            dA = tA * (maxVel + abs(oldVel)) / 2;
        end
    
        distanceTotal = abs(posRef - oldPos + sM*dB);
                    
        tD = maxVel / maxAcc;
        distanceDecelerate = tD * (maxVel) / 2;
        dCV = distanceTotal - (dA + distanceDecelerate);
        tCV = dCV / maxVel;
    
        if (tCV > 0)    % trapezoidal s
            s = 1;
            vT = 0;
        else                % triangular s
            s = 0;
            % Recalculate distances and periods
            if (sM ~= sign(oldVel))  % means brake is needed
                vT = sqrt(maxAcc*(distanceTotal));
                tA = (vT / maxAcc);
                dA = tA * (vT / 2);
            else
                tB = 0;
                dB = 0;
                distanceTotal = abs(posRef - oldPos);      % recalculate total distance
                vT = sqrt(0.5*oldVel^2 + maxAcc*distanceTotal);
                tA = (vT - abs(oldVel)) / maxAcc;
                dA = tA * (vT + abs(oldVel)) / 2;
            end
            tD = vT / maxAcc;
            distanceDecelerate = tD * (vT) / 2;
        end
        timeBrake = tB;
        distanceBrake = dB;
        timeAccelerate = tA;
        distanceAccelerate = dA;
        distanceConstVelocity = dCV;
        timeConstVelocity = tCV;
        timeDecelerate = tD;
        shape = s;
        velTop = vT;
        signM = sM;
        oV = oldVel;
        oP = oldPos;
    end
    
    tB = timeBrake;
    dB = distanceBrake;
    tA = timeAccelerate;
    dA = distanceAccelerate;
    dCV = distanceConstVelocity;
    tCV = timeConstVelocity;
    tD = timeDecelerate;
    s = shape;
    vT = velTop;
    sM = signM;
    time = time + CYCLE_FREQ;
    t = time;
    oV = oldVel;
    oP = oldPos;
end

== matlab function URController/Subsystem/Control System/motionGenerator6/MATLAB Function1 ==
  data: timeBrake input; distanceBrake input; timeAccelerate input; distanceAccelerate input; distanceConstVelocity input; timeConstVelocity input; shape input; velTop input; timeDecelerate input; signM input; deltaTime input; posRef input; pos output; vel output; oldPos input; oldVel input; maxAcc input; maxVel input; acc output
function [pos, vel, acc]   = calculateTrapezoidalProfile(timeBrake, distanceBrake, timeAccelerate, ...
    distanceAccelerate, distanceConstVelocity, timeConstVelocity, shape,  velTop, timeDecelerate, ...
    signM, deltaTime, posRef, oldPos, oldVel, maxAcc, maxVel)
    
    t = deltaTime;
    acc = 0;
    
    if (shape)   % trapezoidal shape
        if (t <= (timeBrake+timeAccelerate))
            pos = oldPos + oldVel*t + signM * 0.5*maxAcc*t^2;
            vel = oldVel + signM * maxAcc*t;
            acc = signM * maxAcc;
        elseif (t > (timeBrake+timeAccelerate) && t < (timeBrake+timeAccelerate+timeConstVelocity))
            pos = oldPos + signM * (-distanceBrake + distanceAccelerate + maxVel*(t-timeBrake-timeAccelerate));
            vel = signM * maxVel;
            % MG.acc = 0;
        elseif (t >= (timeBrake+timeAccelerate+timeConstVelocity) && t < (timeBrake+timeAccelerate+timeConstVelocity+timeDecelerate))
            pos = oldPos + signM * (-distanceBrake + distanceAccelerate + distanceConstVelocity + maxVel*(t-timeBrake-timeAccelerate-timeConstVelocity) - 0.5*maxAcc*(t-timeBrake-timeAccelerate-timeConstVelocity)^2);
            vel = signM * (maxVel - maxAcc*(t-timeBrake-timeAccelerate-timeConstVelocity));
            acc = - signM * maxAcc;
        else
            pos = posRef;
            vel = 0;
            % MG.acc = 0;
        end
    else            % triangular shape
        if (t <= (timeBrake+timeAccelerate))
            pos = oldPos + oldVel*t + signM * 0.5*maxAcc*t^2;
            vel = oldVel + signM * maxAcc*t;
            acc = signM * maxAcc;
        elseif (t > (timeBrake+timeAccelerate) && t < (timeBrake+timeAccelerate+timeDecelerate))
            pos = oldPos + signM * (-distanceBrake + distanceAccelerate + velTop*(t-timeBrake-timeAccelerate) - 0.5*maxAcc*(t-timeBrake-timeAccelerate)^2);
            vel = signM * (velTop - maxAcc*(t-timeBrake-timeAccelerate));
            acc = - signM * maxAcc;
        else
            pos = posRef;
            vel = 0;
            acc = 0;
        end
        
    end

end

== matlab function URController/Subsystem/Kinematic calculator/MATLAB Function2 ==
  data: ori_theta input; theta input; solution output
function solution = solutionSelector(ori_theta, theta)

[~, index] = min(sum(abs(theta - ori_theta), 1));
solution = theta(:, index);    

end

== matlab function URController/MATLAB Function ==
  data: mat4x4 input; pos output; ori output
function [pos, ori] = convertMat2PosRot(mat4x4)
    ori = rotm2eul(mat4x4(1:3, 1:3), "XYZ");
    px = mat4x4(1,4);
    py = mat4x4(2,4);
    pz = mat4x4(3,4);
    pos = [px, py, pz];
end

== matlab function URController/Subsystem/isInitialized ==
  data: u input; y output
function y = isInitialized(u)

s = sum(u);
if s == 0 
    y = 1;
else 
    y = -1;
end
